simulink model "Simu_q2"  (R2018a)
settings: Solver=VariableStepAuto  StartTime=0.0  StopTime=150  RelTol=1e-3
libraries: simulink x2
settings Model: Creator=55479  LastModifiedBy=55479

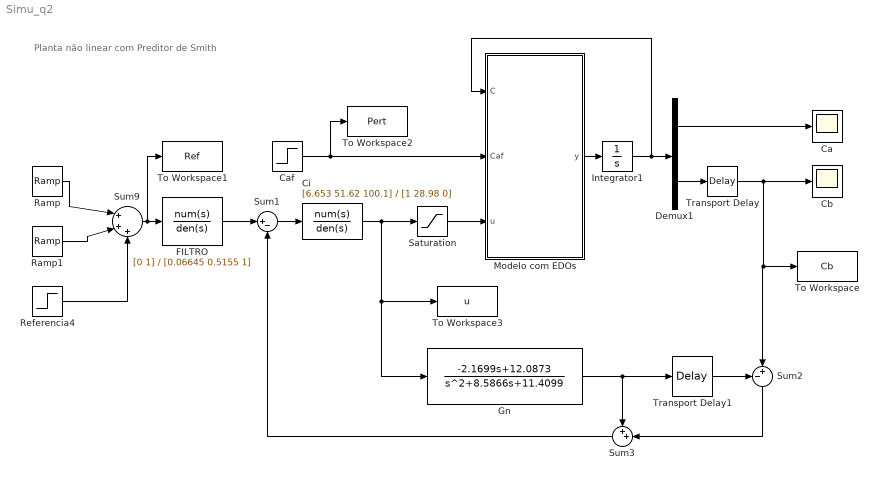
== system Simu_q2 ==
  note: Planta não linear com Preditor de Smith
  "Ca  " : Scope
  Caf : Step  Time=90  Before=5.1  After=5.1  SampleTime=0
  "Cb  " : Scope
  Ci : TransferFcn  Numerator=[6.653 51.62 100.1]  Denominator=[1 28.98 0]
  Demux1 : Demux  Outputs=2
  "FILTRO " : TransferFcn  Numerator=[0 1]  Denominator=[0.06645 0.5155 1]
  Gn : TransferFcn  Numerator=[-2.1699 12.0873]  Denominator="[1 8.5866  11.4099]"
  Integrator1 : Integrator  InitialCondition=[0;0]
  Modelo com EDOs : MATLAB Function  TreatAsAtomicUnit=on
  Ramp : simulink/Sources/Ramp  slope=1.6/10  start=0  InitialOutput=0
  Ramp1 : simulink/Sources/Ramp  slope=-1.6/10  start=10  InitialOutput=0
  Referencia4 : Step  Time=60  After=-0.25  SampleTime=0
  Saturation : Saturate  UpperLimit=10  LowerLimit=0
  Sum1 : Sum  Inputs=|+-
  Sum2 : Sum  Inputs=-+|
  Sum3 : Sum  Inputs=++|
  Sum9 : Sum  Inputs=|+++
  To Workspace : ToWorkspace  VariableName=Cb  SaveFormat=Timeseries  SampleTime=-1
  To Workspace1 : ToWorkspace  VariableName=Ref  SaveFormat=Timeseries  SampleTime=-1
  To Workspace2 : ToWorkspace  VariableName=Pert  SaveFormat=Timeseries  SampleTime=-1
  To Workspace3 : ToWorkspace  VariableName=u  SaveFormat=Timeseries  SampleTime=-1
  Transport Delay : TransportDelay  DelayTime=3
  Transport Delay1 : TransportDelay  DelayTime=3
  wires:
  Referencia4/1 -> Sum9/3
  Ci/1 -> To Workspace3/1, Gn/1, Saturation/1
  Demux1/1 -> "Ca  "/1
  Caf/1 -> To Workspace2/1, Modelo com EDOs/2(Caf)
  Ramp/1 -> Sum9/1
  Sum3/1 -> Sum1/2
  Transport Delay1/1 -> Sum2/1
  Ramp1/1 -> Sum9/2
  Transport Delay/1 -> "Cb  "/1, Sum2/2, To Workspace/1
  Sum2/1 -> Sum3/2
  Sum1/1 -> Ci/1
  "FILTRO "/1 -> Sum1/1
  Integrator1/1 -> Demux1/1, Modelo com EDOs/1(C)
  Demux1/2 -> Transport Delay/1
  Sum9/1 -> To Workspace1/1, "FILTRO "/1
  Gn/1 -> Transport Delay1/1, Sum3/1
  Modelo com EDOs/1(y) -> Integrator1/1
  Saturation/1 -> Modelo com EDOs/3(u)

== matlab function Simu_q2/Modelo com EDOs ==
  data: y output; C input; Caf input; u input
%EDOs das concentracoes dos produtos A e B
function y = fcn(C, Caf, u)

%constantes
k1 = 6.01; %L/min
k2 = 0.8433; %L/min
k3 = 0.1123; %mol/Lmin

%variaveis das concentracoes dos produtos A e B
Ca = C(1);
Cb = C(2);

%EDOs
Ca_d = -k1*Ca - k3*(Ca^2) + (Caf - Ca)*u;
Cb_d =  k1*Ca - k2*Cb - Cb*u;
 
%conjunto das EDOs
y = [Ca_d;Cb_d];
